simulink model "Project_Simulink"  (R2016a)
settings: Solver=FixedStepAuto  StartTime=0.0  StopTime=inf  RelTol=1e-3
libraries: arduinolib x6
settings Model: SimulationMode=external  ExtModeTrigDuration=2  Creator=Nada  LastModifiedBy=Nada
settings OptimizationCC: OptimizeModelRefInitCode=on  LifeSpan=Inf  MaxStackSize=64
settings HardwareCC: ProdBitPerInt=16  ProdBitPerPointer=16  ProdLargestAtomicFloat=None  ProdWordSize=8  ProdHWDeviceType=Atmel->AVR
settings RTWCC: SystemTargetFile=ert.tlc  HardwareBoard=Arduino Uno  TemplateMakefile=ert_default_tmf  GenerateReport=on  Toolchain=Arduino AVR v1.6.1  BuildConfiguration=Faster Runs  IncludeHyperlinkInReport=on  LaunchReport=on  GenerateTraceInfo=on  GenerateTraceReport=on  GenerateTraceReportSl=on  GenerateTraceReportSf=on  GenerateTraceReportEml=on
settings CodeAppCC: ForceParamTrailComments=on  IgnoreCustomStorageClasses=off  OperatorAnnotations=on  SimulinkDataObjDesc=on  SFDataObjDesc=on  MATLABFcnDesc=on  InsertBlockDesc=on  MATLABSourceComments=on
settings ERTTargetCC: SupportContinuousTime=on  SupportVariableSizeSignals=on

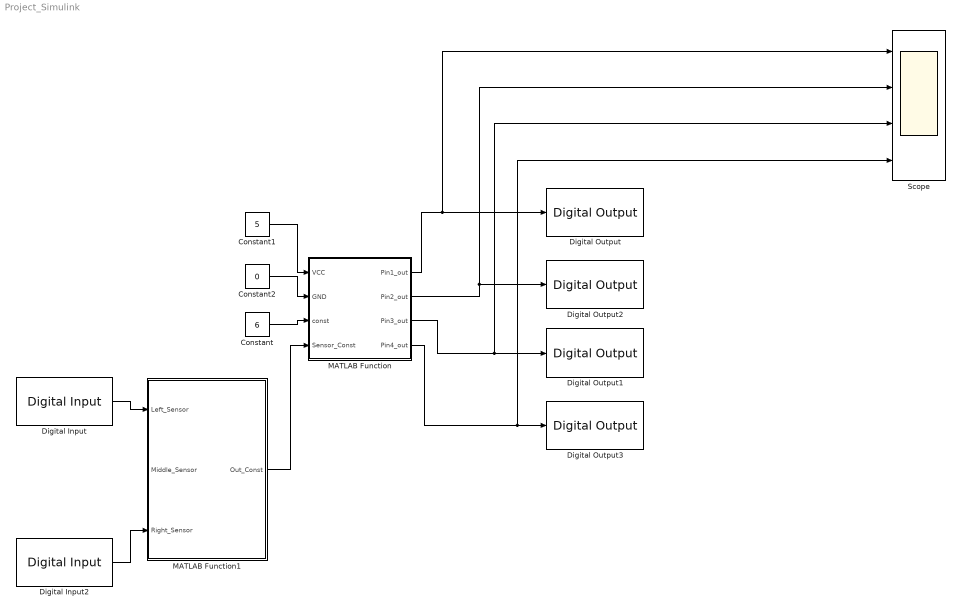
== system Project_Simulink ==
  Constant : Constant  Value=6
  Constant1 : Constant  Value=5
  Constant2 : Constant  Value=0
  Digital Input : arduinolib/Digital Input  pinNumber=3  sampleTime=1  blockPlatform=arduino
  Digital Input2 : arduinolib/Digital Input  pinNumber=5  sampleTime=1  blockPlatform=arduino
  Digital Output : arduinolib/Digital Output  pinNumber=8  blockPlatform=arduino
  Digital Output1 : arduinolib/Digital Output  pinNumber=10  blockPlatform=arduino
  Digital Output2 : arduinolib/Digital Output  pinNumber=9  blockPlatform=arduino
  Digital Output3 : arduinolib/Digital Output  pinNumber=11  blockPlatform=arduino
  MATLAB Function : MATLAB Function  TreatAsAtomicUnit=on
  MATLAB Function1 : MATLAB Function  TreatAsAtomicUnit=on
  Scope : Scope  NumInputPorts=4
  wires:
  MATLAB Function/1(Pin1_out) -> Scope/1, Digital Output/1
  MATLAB Function/2(Pin2_out) -> Scope/2, Digital Output2/1
  MATLAB Function/3(Pin3_out) -> Scope/3, Digital Output1/1
  MATLAB Function/4(Pin4_out) -> Scope/4, Digital Output3/1
  Constant/1 -> MATLAB Function/3(const)
  Constant1/1 -> MATLAB Function/1(VCC)
  Constant2/1 -> MATLAB Function/2(GND)
  Digital Input2/1 -> MATLAB Function1/3(Right_Sensor)
  Digital Input/1 -> MATLAB Function1/1(Left_Sensor)
  MATLAB Function1/1(Out_Const) -> MATLAB Function/4(Sensor_Const)

== matlab function Project_Simulink/MATLAB Function1 ==
  data: Left_Sensor input; Middle_Sensor input; Out_Const output; Right_Sensor input
function Out_Const  = fcn(Left_Sensor,Middle_Sensor,Right_Sensor)
%#codegen
% surface then arduino gets 1 as input 
%and when senses black line arduino gets 0 as input.
if ((Left_Sensor >= 0) && (Middle_Sensor == 1) && (Right_Sensor >= 0)) % forward
    Out_Const=1;
elseif ((Left_Sensor >= 0) && (Middle_Sensor >= 0) && (Right_Sensor == 1)) % Right
    Out_Const=3;
elseif ((Left_Sensor ==1) && (Middle_Sensor >=0) && (Right_Sensor >= 0)) % left
    Out_Const=4;  
else
    Out_Const=7;  
    
end

== matlab function Project_Simulink/MATLAB Function ==
  data: VCC input; Pin1_out output; GND input; const input; Pin2_out output; Pin3_out output; Pin4_out output; Sensor_Const input


function [Pin1_out,Pin2_out,Pin3_out,Pin4_out] = fcn(VCC,GND,const,Sensor_Const)

% Line Follower *******************************

if(const == 6 && Sensor_Const ==1) % forward
    Pin1_out=VCC;
    Pin2_out=GND;
    Pin3_out=VCC;
    Pin4_out=GND;
elseif(const == 6 && Sensor_Const ==3) % right 
    Pin1_out=GND;
    Pin2_out=VCC;
    Pin3_out=GND;
    Pin4_out=GND;
elseif (const == 6 && Sensor_Const ==4) %Left
    Pin1_out=GND;
    Pin2_out=GND;
    Pin3_out=GND;
    Pin4_out=VCC;    
elseif (const == 1) %forward
    Pin1_out=VCC;
    Pin2_out=GND;
    Pin3_out=VCC;
    Pin4_out=GND;
elseif (const == 2) %reverse
    Pin1_out=GND;
    Pin2_out=VCC;
    Pin3_out=GND;
    Pin4_out=VCC;
elseif (const == 3) %right
    Pin1_out=GND;
    Pin2_out=VCC;
    Pin3_out=GND;
    Pin4_out=GND;
elseif (const == 4) %Left
    Pin1_out=GND;
    Pin2_out=GND;
    Pin3_out=GND;
    Pin4_out=VCC;
else    %stop
    Pin1_out=GND;
    Pin2_out=GND;
    Pin3_out=GND;
    Pin4_out=GND;

end
